simulink model "reward_fun"  (R2023b)
settings: Solver=VariableStepAuto  StartTime=0.0  StopTime=10.0  RelTol=1e-3
values from neighbouring files (symbols this model uses):
  alpha_bal_threshold = pi/6    (= 0.523598775598)    [loadQubeParametersB.m]
  B = -100    [loadQubeParametersB.m]
  q11 = 0.166    [loadQubeParametersB.m]
  q22 = 0.5    [loadQubeParametersB.m]
  q33 = 0.01    [loadQubeParametersB.m]
  q44 = 0    [loadQubeParametersB.m]
  r = .0001    (= 0.0001)    [loadQubeParametersB.m]
  theta_max = 3*pi/4    (= 2.35619449019)    [loadQubeParametersB.m]
  Vmax = 10    [loadQubeParametersB.m]
libraries: simulink x3
settings Model: Creator=user  LastModifiedBy=user

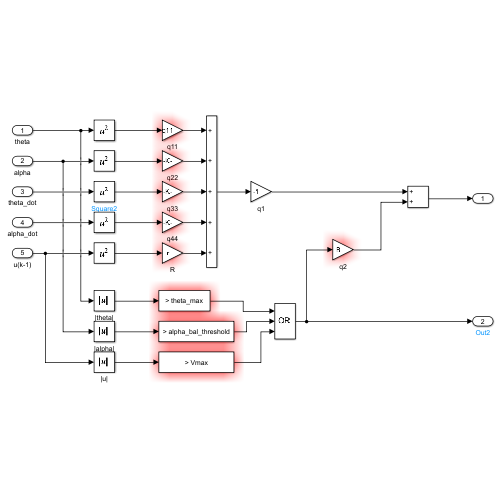
[thumbnail: Simulink's stored preview of the top-level diagram]
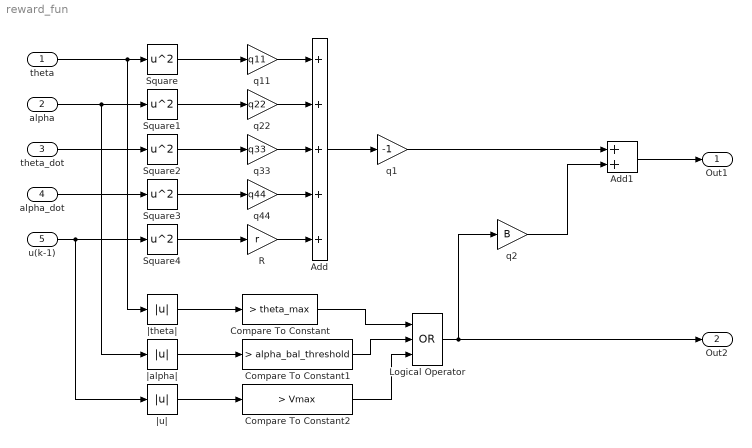
== system reward_fun ==
  theta : Inport
  alpha : Inport  Port=2
  theta_dot : Inport  Port=3
  alpha_dot : Inport  Port=4
  u(k-1) : Inport  Port=5
  Add : Sum  Inputs=+++++
  Add1 : Sum
  Compare To Constant : simulink/Logic and Bit Operations/Compare To Constant  relop=>  const=theta_max  OutDataTypeStr=boolean
  Compare To Constant1 : simulink/Logic and Bit Operations/Compare To Constant  relop=>  const=alpha_bal_threshold  OutDataTypeStr=boolean
  Compare To Constant2 : simulink/Logic and Bit Operations/Compare To Constant  relop=>  const=Vmax  OutDataTypeStr=boolean
  Logical Operator : Logic  Operator=OR  Inputs=3  AllPortsSameDT=off  OutDataTypeStr=boolean
  R : Gain  Gain=r
  Square{,1..4} (5 alike) : Math  Operator=square
  q1 : Gain  Gain=-1
  q11 : Gain  Gain=q11
  q2 : Gain  Gain=B
  q22 : Gain  Gain=q22
  q33 : Gain  Gain=q33
  q44 : Gain  Gain=q44
  |alpha| : Abs  SaturateOnIntegerOverflow=off
  |theta| : Abs  SaturateOnIntegerOverflow=off
  |u| : Abs  SaturateOnIntegerOverflow=off
  Out1 : Outport
  Out2 : Outport  Port=2
  wires:
  u(k-1)/1 -> |u|/1, Square4/1
  alpha_dot/1 -> Square3/1
  theta_dot/1 -> Square2/1
  alpha/1 -> |alpha|/1, Square1/1
  theta/1 -> |theta|/1, Square/1
  Square/1 -> q11/1
  Square1/1 -> q22/1
  Square2/1 -> q33/1
  Square3/1 -> q44/1
  Square4/1 -> R/1
  q11/1 -> Add/1
  q22/1 -> Add/2
  q33/1 -> Add/3
  q44/1 -> Add/4
  R/1 -> Add/5
  Add/1 -> q1/1
  q1/1 -> Add1/1
  |theta|/1 -> Compare To Constant/1
  |alpha|/1 -> Compare To Constant1/1
  |u|/1 -> Compare To Constant2/1
  Compare To Constant2/1 -> Logical Operator/3
  Compare To Constant1/1 -> Logical Operator/2
  Compare To Constant/1 -> Logical Operator/1
  Logical Operator/1 -> Out2/1, q2/1
  q2/1 -> Add1/2
  Add1/1 -> Out1/1
